simulink model "PubIfDecisionLM_MDL"  (R2020b)
settings: configuration reference "DspaceConfig" (kept outside this file)
PostLoadFcn:
  | if any(exist('dsrtsu_mdlpostloadfcn', 'file') ~= 0), dsrtsu_mdlpostloadfcn('Execute', bdroot); end
InitFcn:
  | , if any(exist('dsmpb_private', 'file') ~= 0), dsmpb_private('dsmpb_mdlclblib', 'Init', bdroot); end,
undefined symbols (not defined in the file or in its folder): OFM_OBJ_FUSIONTYPE_E, OFM_OBJ_MOVINGSTATE_E, OFM_OBJ_ORIENTATION_E, OFM_OBJ_TYPE_E, P_LM_Cyc, P_LM_EMLHistKapRcdBufSize, P_LM_EMLHistTrajBaseDis, P_LM_EMLHistTrajPNum, P_LM_EMLKapCorrMaxThre, P_LM_EMLMinKapThre, P_LM_EMLPathDisDiffThre, P_LM_EMLQuaFiltPar, P_LM_EMLTurnActKapThre, P_LM_EMLValidQuaThre, P_LM_FntPath1Disgap, P_LM_FntPath1MinDis, P_LM_FntPath1Timegap, P_LM_FntPath2Disgap, P_LM_FntPath2MinDis, P_LM_FntPath2Timegap, P_LM_FntPath3Disgap, P_LM_FntPath3MinDis, P_LM_FntPath3Timegap, P_LM_FusBLParFiltP, P_LM_FusEVDifC2Thre, P_LM_FusEVOPath1AllVSLDisThre, P_LM_FusEVOPath1AllVSLLostNumThre, P_LM_FusEVOPath1AllVSLQuaThre, P_LM_FusEVOPath1OTLFacNLC, P_LM_FusOTLQuaThre, P_LM_FusOTLSW, P_LM_FusParC0Index, P_LM_FusParC1Index, P_LM_FusParC2Index, P_LM_FusParC3Index, P_LM_FusVSLQuaThre, P_LM_FusVSLSW, P_LM_FusVSLValidSteerWheerAngThre, P_LM_FusVSLValidVxvThre, P_LM_LaneWidth, P_LM_OTLBufTPInfoEvaFactor, P_LM_OTLObjNum, P_LM_OTLObjSelectAgeThre, P_LM_OTLObjSelectDxAssessVx, P_LM_OTLObjSelectDxThre, P_LM_OTLObjSelectVxThre, P_LM_OTLObjSelectVyAssessDx, P_LM_OTLObjSelectVyThre, P_LM_OTLTrajPntBaseDis, P_LM_OTLTrajStdThre, P_LM_VSLAvailLineNum, P_LM_VSLBLSDiffThre, P_LM_VSLBLSDisRatio, P_LM_VSLFusBLParFiltP_C1, P_LM_VSLFusBLParFiltP_C2, P_LM_VSLFusBLParFiltP_C3, P_LM_VSLFusBLParFiltP_Quality, P_LM_VSLHistTrajBaseDis, P_LM_VSLHistTrajPNum, P_LM_VSLLCC0diff ... (+18)
libraries: simulink x145, LM_LIB x43
(part 23 of 24)

== matlab function PubIfDecisionLM_MDL/Subsystem2/LM_OTL/LM_OTL_MovObjTrajFit/LM_OTL_TrajFit/MATLAB Function3 ==
  data: LM_OTLBufL1DxVect input; LM_OTLBufL1DyVect input; LM_OTLBufL2DxVect input; LM_OTLBufL2DyVect input; LM_OTLBufE1DxVect input; LM_OTLBufE1DyVect input; LM_OTLBufE2DxVect input; LM_OTLBufE2DyVect input; LM_OTLBufR1DxVect input; LM_OTLBufR1DyVect input; LM_OTLBufR2DxVect input; LM_OTLBufR2DyVect input; LM_OTLBufL1SPPos input; LM_OTLBufL2SPPos input; LM_OTLBufE1SPPos input; LM_OTLBufE2SPPos input; LM_OTLBufR1SPPos input; LM_OTLBufR2SPPos input; LM_OTLBufL1LastSPPos input; LM_OTLBufL2LastSPPos input; LM_OTLBufE1LastSPPos input; LM_OTLBufE2LastSPPos input; LM_OTLBufR1LastSPPos input; LM_OTLBufR2LastSPPos input; LM_OTLBufL1PNum input; LM_OTLBufL2PNum input; LM_OTLBufE1PNum input; LM_OTLBufE2PNum input; LM_OTLBufR1PNum input; LM_OTLBufR2PNum input; LM_OTLBufL1LastPNum input; LM_OTLBufL2LastPNum input; LM_OTLBufE1LastPNum input; LM_OTLBufE2LastPNum input; LM_OTLBufR1LastPNum input; LM_OTLBufR2LastPNum input; LM_OTLBufL1Flg input; LM_OTLBufL2Flg input; LM_OTLBufE1Flg input; LM_OTLBufE2Flg input; LM_OTLBufR1Flg input; LM_OTLBufR2Flg input; LM_OTLBufL1LastFlg input; LM_OTLBufL2LastFlg input; LM_OTLBufE1LastFlg input; LM_OTLBufE2LastFlg input; LM_OTLBufR1LastFlg input; LM_OTLBufR2LastFlg input; LM_OTLBufL1Offset input; LM_OTLBufL2Offset input; LM_OTLBufE1Offset input; LM_OTLBufE2Offset input; LM_OTLBufR1Offset input; LM_OTLBufR2Offset input; LM_OTLBufL1LastOffset input; LM_OTLBufL2LastOffset input; LM_OTLBufE1LastOffset input; LM_OTLBufE2LastOffset input; LM_OTLBufR1LastOffset input; LM_OTLBufR2LastOffset input; LM_OTLBufResampeFntPathDxInfo output; LM_OTLBufResampeFntPathDyInfo output
function [LM_OTLBufResampeFntPathDxInfo,LM_OTLBufResampeFntPathDyInfo] = fcn(LM_OTLBufL1DxVect,LM_OTLBufL1DyVect,LM_OTLBufL2DxVect,LM_OTLBufL2DyVect,LM_OTLBufE1DxVect,LM_OTLBufE1DyVect,LM_OTLBufE2DxVect,LM_OTLBufE2DyVect,LM_OTLBufR1DxVect,LM_OTLBufR1DyVect,LM_OTLBufR2DxVect,LM_OTLBufR2DyVect,...
                                                              LM_OTLBufL1SPPos,LM_OTLBufL2SPPos,LM_OTLBufE1SPPos,LM_OTLBufE2SPPos,LM_OTLBufR1SPPos,LM_OTLBufR2SPPos,LM_OTLBufL1LastSPPos,LM_OTLBufL2LastSPPos,LM_OTLBufE1LastSPPos,LM_OTLBufE2LastSPPos,LM_OTLBufR1LastSPPos,LM_OTLBufR2LastSPPos,...
                                                              LM_OTLBufL1PNum,LM_OTLBufL2PNum,LM_OTLBufE1PNum,LM_OTLBufE2PNum,LM_OTLBufR1PNum,LM_OTLBufR2PNum,LM_OTLBufL1LastPNum,LM_OTLBufL2LastPNum,LM_OTLBufE1LastPNum,LM_OTLBufE2LastPNum,LM_OTLBufR1LastPNum,LM_OTLBufR2LastPNum,...
                                                              LM_OTLBufL1Flg,LM_OTLBufL2Flg,LM_OTLBufE1Flg,LM_OTLBufE2Flg,LM_OTLBufR1Flg,LM_OTLBufR2Flg,LM_OTLBufL1LastFlg,LM_OTLBufL2LastFlg,LM_OTLBufE1LastFlg,LM_OTLBufE2LastFlg,LM_OTLBufR1LastFlg,LM_OTLBufR2LastFlg,...
                                                              LM_OTLBufL1Offset,LM_OTLBufL2Offset,LM_OTLBufE1Offset,LM_OTLBufE2Offset,LM_OTLBufR1Offset,LM_OTLBufR2Offset,LM_OTLBufL1LastOffset,LM_OTLBufL2LastOffset,LM_OTLBufE1LastOffset,LM_OTLBufE2LastOffset,LM_OTLBufR1LastOffset,LM_OTLBufR2LastOffset)
                                                               
%第一段车道车道线采样
%初始化基本参数
P_LM_OTLBufResampPNum = uint8(40);
P_LM_OTLBufResampSPPos = single(0);
P_LM_OTLBufResampBaseDis = single(2);
% output initial                                                           
LM_OTLBufResampeFntPathDxInfo = single(zeros(1,80));
LM_OTLBufResampeFntPathDyInfo = single(zeros(1,80));
%初始化各buffer轨迹点索引位置  
t_bufl1index = uint8(0);
t_bufl2index = uint8(0);
t_bufe1index = uint8(0);
t_bufe2index = uint8(0);
t_bufr1index = uint8(0);
t_bufr2index = uint8(0);
t_bufl1lastindex = uint8(0);
t_bufl2lastindex = uint8(0);
t_bufe1lastindex = uint8(0);
t_bufe2lastindex = uint8(0);
t_bufr1lastindex = uint8(0);
t_bufr2lastindex = uint8(0);
%第一段车道车道线采样
for i = 1:P_LM_OTLBufResampPNum
    temp1 = (single(i-1))*P_LM_OTLBufResampBaseDis + P_LM_OTLBufResampSPPos;
    temp2 = (single(i))*P_LM_OTLBufResampBaseDis + P_LM_OTLBufResampSPPos;
    %初始化该区间范围内有效轨迹点个数
    t_tpnum = uint8(0);
    t_tpdxsum = single(0);
    t_tpdysum = single(0);
    %判断BufL1前目标是否存在该区间的轨迹点
    if LM_OTLBufL1LastFlg(1) ~= 0
        if t_bufl1lastindex < LM_OTLBufL1LastPNum(1)
            t_index = t_bufl1lastindex + LM_OTLBufL1LastSPPos(1);
            if t_index > 80
                t_index = t_index - uint8(80);
            end
            t_tpdx = LM_OTLBufL1DxVect(t_index);
            t_tpdy = LM_OTLBufL1DyVect(t_index)-LM_OTLBufL1LastOffset(1);
            if t_tpdx >= temp1  && t_tpdx < temp2
                t_tpnum = t_tpnum +uint8(1);
                t_tpdxsum = t_tpdxsum + t_tpdx;
                t_tpdysum = t_tpdysum + t_tpdy;
                t_bufl1lastindex = t_bufl1lastindex +uint8(1);
            end
        end
    end
    %判断BufL1当前目标是否存在该区间的轨迹点
    if LM_OTLBufL1Flg(1) ~= 0
        if t_bufl1index < LM_OTLBufL1PNum(1)
            t_index = t_bufl1index + LM_OTLBufL1SPPos(1);
            if t_index > 80
                t_index = t_index - uint8(80);
            end
            t_tpdx = LM_OTLBufL1DxVect(t_index);
            t_tpdy = LM_OTLBufL1DyVect(t_index)-LM_OTLBufL1Offset(1);
            if t_tpdx >= temp1  && t_tpdx < temp2
                t_tpnum = t_tpnum +uint8(1);
                t_tpdxsum = t_tpdxsum + t_tpdx;
                t_tpdysum = t_tpdysum + t_tpdy;
                t_bufl1index = t_bufl1index +uint8(1);
            end
        end
    end
    %判断BufL2前目标是否存在该区间的轨迹点
    if LM_OTLBufL2LastFlg(1) ~= 0
        if t_bufl2lastindex < LM_OTLBufL2LastPNum(1)
            t_index = t_bufl2lastindex + LM_OTLBufL2LastSPPos(1);
            if t_index > 80
                t_index = t_index - uint8(80);
            end
            t_tpdx = LM_OTLBufL2DxVect(t_index);
            t_tpdy = LM_OTLBufL2DyVect(t_index)-LM_OTLBufL2LastOffset(1);
            if t_tpdx >= temp1  && t_tpdx < temp2 
                t_tpnum = t_tpnum +uint8(1);
                t_tpdxsum = t_tpdxsum + t_tpdx;
                t_tpdysum = t_tpdysum + t_tpdy;
                t_bufl2lastindex = t_bufl2lastindex +uint8(1);
            end
        end
    end
    %判断BufL2当前目标是否存在该区间的轨迹点
    if LM_OTLBufL2Flg(1) ~= 0
        if t_bufl2index < LM_OTLBufL2PNum(1)
            t_index = t_bufl2index + LM_OTLBufL2SPPos(1);
            if t_index > 80
                t_index = t_index - uint8(80);
            end
            t_tpdx = LM_OTLBufL2DxVect(t_index);
            t_tpdy = LM_OTLBufL2DyVect(t_index)-LM_OTLBufL2Offset(1);
            if t_tpdx >= temp1  && t_tpdx < temp2 
                t_tpnum = t_tpnum +uint8(1);
                t_tpdxsum = t_tpdxsum + t_tpdx;
                t_tpdysum = t_tpdysum + t_tpdy;
                t_bufl2index = t_bufl2index +uint8(1);
            end
        end
    end
    %判断BufE1前目标是否存在该区间的轨迹点
    if LM_OTLBufE1LastFlg(1) ~= 0
        if t_bufe1lastindex < LM_OTLBufE1LastPNum(1)
            t_index = t_bufe1lastindex + LM_OTLBufE1LastSPPos(1);
            if t_index > 80
                t_index = t_index - uint8(80);
            end
            t_tpdx = LM_OTLBufE1DxVect(t_index);
            t_tpdy = LM_OTLBufE1DyVect(t_index)-LM_OTLBufE1LastOffset(1);
            if t_tpdx >= temp1  && t_tpdx < temp2 
                t_tpnum = t_tpnum +uint8(1);
                t_tpdxsum = t_tpdxsum + t_tpdx;
                t_tpdysum = t_tpdysum + t_tpdy;
                t_bufe1lastindex = t_bufe1lastindex +uint8(1);
            end
        end
    end
    %判断BufE1当前目标是否存在该区间的轨迹点
    if LM_OTLBufE1Flg(1) ~= 0
        if t_bufe1index < LM_OTLBufE1PNum(1)
            t_index = t_bufe1index + LM_OTLBufE1SPPos(1);
            if t_index > 80
                t_index = t_index - uint8(80);
            end
            t_tpdx = LM_OTLBufE1DxVect(t_index);
            t_tpdy = LM_OTLBufE1DyVect(t_index)-LM_OTLBufE1Offset(1);
            if t_tpdx >= temp1  && t_tpdx < temp2 
                t_tpnum = t_tpnum +uint8(1);
                t_tpdxsum = t_tpdxsum + t_tpdx;
                t_tpdysum = t_tpdysum + t_tpdy;
                t_bufe1index = t_bufe1index +uint8(1);
            end
        end
    end
    %判断BufE2前目标是否存在该区间的轨迹点
    if LM_OTLBufE2LastFlg(1) ~= 0
        if t_bufe2lastindex < LM_OTLBufE2LastPNum(1)
            t_index = t_bufe2lastindex + LM_OTLBufE2LastSPPos(1);
            if t_index > 80
                t_index = t_index - uint8(80);
            end
            t_tpdx = LM_OTLBufE2DxVect(t_index);
            t_tpdy = LM_OTLBufE2DyVect(t_index)-LM_OTLBufE2LastOffset(1);
            if t_tpdx >= temp1 && t_tpdx < temp2 
                t_tpnum = t_tpnum +uint8(1);
                t_tpdxsum = t_tpdxsum + t_tpdx;
                t_tpdysum = t_tpdysum + t_tpdy;
                t_bufe2lastindex = t_bufe2lastindex +uint8(1);
            end
        end
    end
    %判断BufE2当前目标是否存在该区间的轨迹点
    if LM_OTLBufE2Flg(1) ~= 0
        if t_bufe2index < LM_OTLBufE2PNum(1)
            t_index = t_bufe2index + LM_OTLBufE2SPPos(1);
            if t_index > 80
                t_index = t_index - uint8(80);
            end
            t_tpdx = LM_OTLBufE2DxVect(t_index);
            t_tpdy = LM_OTLBufE2DyVect(t_index)-LM_OTLBufE2Offset(1);
            if t_tpdx >= temp1  && t_tpdx < temp2 
                t_tpnum = t_tpnum +uint8(1);
                t_tpdxsum = t_tpdxsum + t_tpdx;
                t_tpdysum = t_tpdysum + t_tpdy;
                t_bufe2index = t_bufe2index +uint8(1);
            end
        end
    end
    %判断BufR1前目标否存在该区间的轨迹点
    if LM_OTLBufR1LastFlg(1) ~= 0
        if t_bufr1lastindex < LM_OTLBufR1LastPNum(1)
            t_index = t_bufr1lastindex +  LM_OTLBufR1LastSPPos(1);
            if t_index > 80
                t_index = t_index - uint8(80);
            end
            t_tpdx = LM_OTLBufR1DxVect(t_index);
            t_tpdy = LM_OTLBufR1DyVect(t_index)-LM_OTLBufR1LastOffset(1);
            if t_tpdx >= temp1  && t_tpdx < temp2 
                t_tpnum = t_tpnum +uint8(1);
                t_tpdxsum = t_tpdxsum + t_tpdx;
                t_tpdysum = t_tpdysum + t_tpdy;
                t_bufr1lastindex = t_bufr1lastindex +uint8(1);
            end
        end
    end
    %判断BufR1当前目标否存在该区间的轨迹点
    if LM_OTLBufR1Flg(1) ~= 0
        if t_bufr1index < LM_OTLBufR1PNum(1)
            t_index = t_bufr1index +  LM_OTLBufR1SPPos(1);
            if t_index > 80
                t_index = t_index - uint8(80);
            end
            t_tpdx = LM_OTLBufR1DxVect(t_index);
            t_tpdy = LM_OTLBufR1DyVect(t_index)-LM_OTLBufR1Offset(1);
            if t_tpdx >= temp1  && t_tpdx < temp2 
                t_tpnum = t_tpnum +uint8(1);
                t_tpdxsum = t_tpdxsum + t_tpdx;
                t_tpdysum = t_tpdysum + t_tpdy;
                t_bufr1index = t_bufr1index +uint8(1);
            end
        end
    end
    %判断BufR2前目标是否存在该区间的轨迹点
    if LM_OTLBufR2LastFlg(1) ~= 0
        if t_bufr2lastindex < LM_OTLBufR2LastPNum(1)
            t_index = t_bufr2lastindex + LM_OTLBufR2LastSPPos(1);
            if t_index > 80
                t_index = t_index - uint8(80);
            end
            t_tpdx = LM_OTLBufR2DxVect(t_index);
            t_tpdy = LM_OTLBufR2DyVect(t_index)-LM_OTLBufR2LastOffset(1);
            if t_tpdx >= temp1  && t_tpdx < temp2 
                t_tpnum = t_tpnum +uint8(1);
                t_tpdxsum = t_tpdxsum + t_tpdx;
                t_tpdysum = t_tpdysum + t_tpdy;
                t_bufr2lastindex = t_bufr2lastindex +uint8(1);
            end
        end
    end
    %判断BufR2当前目标是否存在该区间的轨迹点
    if LM_OTLBufR2Flg(1) ~= 0
        if t_bufr2index < LM_OTLBufR2PNum(1)
            t_index = t_bufr2index + LM_OTLBufR2SPPos(1);
            if t_index > 80
                t_index = t_index - uint8(80);
            end
            t_tpdx = LM_OTLBufR2DxVect(t_index);
            t_tpdy = LM_OTLBufR2DyVect(t_index)-LM_OTLBufR2Offset(1);
            if t_tpdx >= temp1  && t_tpdx < temp2 
                t_tpnum = t_tpnum +uint8(1);
                t_tpdxsum = t_tpdxsum + t_tpdx;
                t_tpdysum = t_tpdysum + t_tpdy;
                t_bufr2index = t_bufr2index +uint8(1);
            end
        end
    end
    if t_tpnum ~= 0
        t_tpdx = t_tpdxsum / single(t_tpnum);
        t_tpdy = t_tpdysum / single(t_tpnum);
    else
        t_tpdx = single(0);
        t_tpdy = single(0);
    end
    LM_OTLBufResampeFntPathDxInfo(i) = t_tpdx;
    LM_OTLBufResampeFntPathDyInfo(i) = t_tpdy;
end
%第二段车道车道线采样
%初始化基本参数
P_LM_OTLBufResampPNum = uint8(40);
P_LM_OTLBufResampSPPos = single(35);
P_LM_OTLBufResampBaseDis = single(2);
%初始化各buffer轨迹点索引位置  
t_bufl1index = uint8(0);
t_bufl2index = uint8(0);
t_bufe1index = uint8(0);
t_bufe2index = uint8(0);
t_bufr1index = uint8(0);
t_bufr2index = uint8(0);
t_bufl1lastindex = uint8(0);
t_bufl2lastindex = uint8(0);
t_bufe1lastindex = uint8(0);
t_bufe2lastindex = uint8(0);
t_bufr1lastindex = uint8(0);
t_bufr2lastindex = uint8(0);

for i = 1:P_LM_OTLBufResampPNum
    temp1 = (single(i-1))*P_LM_OTLBufResampBaseDis + P_LM_OTLBufResampSPPos;
    temp2 = (single(i))*P_LM_OTLBufResampBaseDis + P_LM_OTLBufResampSPPos;
    %初始化该区间范围内有效轨迹点个数
    t_tpnum = uint8(0);
    t_tpdxsum = single(0);
    t_tpdysum = single(0);
    %判断BufL1前目标是否存在该区间的轨迹点
    if LM_OTLBufL1LastFlg(2) ~= 0
        if t_bufl1lastindex < LM_OTLBufL1LastPNum(2)
            t_index = t_bufl1lastindex + LM_OTLBufL1LastSPPos(2);
            if t_index > 80
                t_index = t_index - uint8(80);
            end
            t_tpdx = LM_OTLBufL1DxVect(t_index);
            t_tpdy = LM_OTLBufL1DyVect(t_index)-LM_OTLBufL1LastOffset(2);
            if t_tpdx >= temp1  && t_tpdx < temp2
                t_tpnum = t_tpnum +uint8(1);
                t_tpdxsum = t_tpdxsum + t_tpdx;
                t_tpdysum = t_tpdysum + t_tpdy;
                t_bufl1lastindex = t_bufl1lastindex +uint8(1);
            end
        end
    end
    %判断BufL1当前目标是否存在该区间的轨迹点
    if LM_OTLBufL1Flg(2) ~= 0
        if t_bufl1index < LM_OTLBufL1PNum(2)
            t_index = t_bufl1index + LM_OTLBufL1SPPos(2);
            if t_index > 80
                t_index = t_index - uint8(80);
            end
            t_tpdx = LM_OTLBufL1DxVect(t_index);
            t_tpdy = LM_OTLBufL1DyVect(t_index)-LM_OTLBufL1Offset(2);
            if t_tpdx >= temp1  && t_tpdx < temp2
                t_tpnum = t_tpnum +uint8(1);
                t_tpdxsum = t_tpdxsum + t_tpdx;
                t_tpdysum = t_tpdysum + t_tpdy;
                t_bufl1index = t_bufl1index +uint8(1);
            end
        end
    end
    %判断BufL2前目标是否存在该区间的轨迹点
    if LM_OTLBufL2LastFlg(2) ~= 0
        if t_bufl2lastindex < LM_OTLBufL2LastPNum(2)
            t_index = t_bufl2lastindex + LM_OTLBufL2LastSPPos(2);
            if t_index > 80
                t_index = t_index - uint8(80);
            end
            t_tpdx = LM_OTLBufL2DxVect(t_index);
            t_tpdy = LM_OTLBufL2DyVect(t_index)-LM_OTLBufL2LastOffset(2);
            if t_tpdx >= temp1  && t_tpdx < temp2 
                t_tpnum = t_tpnum +uint8(1);
                t_tpdxsum = t_tpdxsum + t_tpdx;
                t_tpdysum = t_tpdysum + t_tpdy;
                t_bufl2lastindex = t_bufl2lastindex +uint8(1);
            end
        end
    end
    %判断BufL2当前目标是否存在该区间的轨迹点
    if LM_OTLBufL2Flg(2) ~= 0
        if t_bufl2index < LM_OTLBufL2PNum(2)
            t_index = t_bufl2index + LM_OTLBufL2SPPos(2);
            if t_index > 80
                t_index = t_index - uint8(80);
            end
            t_tpdx = LM_OTLBufL2DxVect(t_index);
            t_tpdy = LM_OTLBufL2DyVect(t_index)-LM_OTLBufL2Offset(2);
            if t_tpdx >= temp1  && t_tpdx < temp2 
                t_tpnum = t_tpnum +uint8(1);
                t_tpdxsum = t_tpdxsum + t_tpdx;
                t_tpdysum = t_tpdysum + t_tpdy;
                t_bufl2index = t_bufl2index +uint8(1);
            end
        end
    end
    %判断BufE1前目标是否存在该区间的轨迹点
    if LM_OTLBufE1LastFlg(2) ~= 0
        if t_bufe1lastindex < LM_OTLBufE1LastPNum(2)
            t_index = t_bufe1lastindex + LM_OTLBufE1LastSPPos(2);
            if t_index > 80
                t_index = t_index - uint8(80);
            end
            t_tpdx = LM_OTLBufE1DxVect(t_index);
            t_tpdy = LM_OTLBufE1DyVect(t_index)-LM_OTLBufE1LastOffset(2);
            if t_tpdx >= temp1  && t_tpdx < temp2 
                t_tpnum = t_tpnum +uint8(1);
                t_tpdxsum = t_tpdxsum + t_tpdx;
                t_tpdysum = t_tpdysum + t_tpdy;
                t_bufe1lastindex = t_bufe1lastindex +uint8(1);
            end
        end
    end
    %判断BufE1当前目标是否存在该区间的轨迹点
    if LM_OTLBufE1Flg(2) ~= 0
        if t_bufe1index < LM_OTLBufE1PNum(2)
            t_index = t_bufe1index + LM_OTLBufE1SPPos(2);
            if t_index > 80
                t_index = t_index - uint8(80);
            end
            t_tpdx = LM_OTLBufE1DxVect(t_index);
            t_tpdy = LM_OTLBufE1DyVect(t_index)-LM_OTLBufE1Offset(2);
            if t_tpdx >= temp1  && t_tpdx < temp2 
                t_tpnum = t_tpnum +uint8(1);
                t_tpdxsum = t_tpdxsum + t_tpdx;
                t_tpdysum = t_tpdysum + t_tpdy;
                t_bufe1index = t_bufe1index +uint8(1);
            end
        end
    end
    %判断BufE2前目标是否存在该区间的轨迹点
    if LM_OTLBufE2LastFlg(2) ~= 0
        if t_bufe2lastindex < LM_OTLBufE2LastPNum(2)
            t_index = t_bufe2lastindex + LM_OTLBufE2LastSPPos(2);
            if t_index > 80
                t_index = t_index - uint8(80);
            end
            t_tpdx = LM_OTLBufE2DxVect(t_index);
            t_tpdy = LM_OTLBufE2DyVect(t_index)-LM_OTLBufE2LastOffset(2);
            if t_tpdx >= temp1 && t_tpdx < temp2 
                t_tpnum = t_tpnum +uint8(1);
                t_tpdxsum = t_tpdxsum + t_tpdx;
                t_tpdysum = t_tpdysum + t_tpdy;
                t_bufe2lastindex = t_bufe2lastindex +uint8(1);
            end
        end
    end
    %判断BufE2当前目标是否存在该区间的轨迹点
    if LM_OTLBufE2Flg(2) ~= 0
        if t_bufe2index < LM_OTLBufE2PNum(2)
            t_index = t_bufe2index + LM_OTLBufE2SPPos(2);
            if t_index > 80
                t_index = t_index - uint8(80);
            end
            t_tpdx = LM_OTLBufE2DxVect(t_index);
            t_tpdy = LM_OTLBufE2DyVect(t_index)-LM_OTLBufE2Offset(2);
            if t_tpdx >= temp1  && t_tpdx < temp2 
                t_tpnum = t_tpnum +uint8(1);
                t_tpdxsum = t_tpdxsum + t_tpdx;
                t_tpdysum = t_tpdysum + t_tpdy;
                t_bufe2index = t_bufe2index +uint8(1);
            end
        end
    end
    %判断BufR1前目标否存在该区间的轨迹点
    if LM_OTLBufR1LastFlg(2) ~= 0
        if t_bufr1lastindex < LM_OTLBufR1LastPNum(2)
            t_index = t_bufr1lastindex +  LM_OTLBufR1LastSPPos(2);
            if t_index > 80
                t_index = t_index - uint8(80);
            end
            t_tpdx = LM_OTLBufR1DxVect(t_index);
            t_tpdy = LM_OTLBufR1DyVect(t_index)-LM_OTLBufR1LastOffset(2);
            if t_tpdx >= temp1  && t_tpdx < temp2 
                t_tpnum = t_tpnum +uint8(1);
                t_tpdxsum = t_tpdxsum + t_tpdx;
                t_tpdysum = t_tpdysum + t_tpdy;
                t_bufr1lastindex = t_bufr1lastindex +uint8(1);
            end
        end
    end
    %判断BufR1当前目标否存在该区间的轨迹点
    if LM_OTLBufR1Flg(2) ~= 0
        if t_bufr1index < LM_OTLBufR1PNum(2)
            t_index = t_bufr1index +  LM_OTLBufR1SPPos(2);
            if t_index > 80
                t_index = t_index - uint8(80);
            end
            t_tpdx = LM_OTLBufR1DxVect(t_index);
            t_tpdy = LM_OTLBufR1DyVect(t_index)-LM_OTLBufR1Offset(2);
            if t_tpdx >= temp1  && t_tpdx < temp2 
                t_tpnum = t_tpnum +uint8(1);
                t_tpdxsum = t_tpdxsum + t_tpdx;
                t_tpdysum = t_tpdysum + t_tpdy;
                t_bufr1index = t_bufr1index +uint8(1);
            end
        end
    end
    %判断BufR2前目标是否存在该区间的轨迹点
    if LM_OTLBufR2LastFlg(2) ~= 0
        if t_bufr2lastindex < LM_OTLBufR2LastPNum(2)
            t_index = t_bufr2lastindex + LM_OTLBufR2LastSPPos(2);
            if t_index > 80
                t_index = t_index - uint8(80);
            end
            t_tpdx = LM_OTLBufR2DxVect(t_index);
            t_tpdy = LM_OTLBufR2DyVect(t_index)-LM_OTLBufR2LastOffset(2);
            if t_tpdx >= temp1  && t_tpdx < temp2 
                t_tpnum = t_tpnum +uint8(1);
                t_tpdxsum = t_tpdxsum + t_tpdx;
                t_tpdysum = t_tpdysum + t_tpdy;
                t_bufr2lastindex = t_bufr2lastindex +uint8(1);
            end
        end
    end
    %判断BufR2当前目标是否存在该区间的轨迹点
    if LM_OTLBufR2Flg(2) ~= 0
        if t_bufr2index < LM_OTLBufR2PNum(2)
            t_index = t_bufr2index + LM_OTLBufR2SPPos(2);
            if t_index > 80
                t_index = t_index - uint8(80);
            end
            t_tpdx = LM_OTLBufR2DxVect(t_index);
            t_tpdy = LM_OTLBufR2DyVect(t_index)-LM_OTLBufR2Offset(2);
            if t_tpdx >= temp1  && t_tpdx < temp2 
                t_tpnum = t_tpnum +uint8(1);
                t_tpdxsum = t_tpdxsum + t_tpdx;
                t_tpdysum = t_tpdysum + t_tpdy;
                t_bufr2index = t_bufr2index +uint8(1);
            end
        end
    end
    if t_tpnum ~= 0
        t_tpdx = t_tpdxsum / single(t_tpnum);
        t_tpdy = t_tpdysum / single(t_tpnum);
    else
        t_tpdx = single(0);
        t_tpdy = single(0);
    end
    if t_tpdx~=0
        index=uint8(ceil(0.5*t_tpdx)+1);
        LM_OTLBufResampeFntPathDxInfo(index) = t_tpdx;
        LM_OTLBufResampeFntPathDyInfo(index) = t_tpdy;
    end
end
%第三段车道车道线采样
%初始化基本参数
P_LM_OTLBufResampPNum = uint8(40);
P_LM_OTLBufResampSPPos = single(70);
P_LM_OTLBufResampBaseDis = single(2);
%初始化各buffer轨迹点索引位置  
t_bufl1index = uint8(0);
t_bufl2index = uint8(0);
t_bufe1index = uint8(0);
t_bufe2index = uint8(0);
t_bufr1index = uint8(0);
t_bufr2index = uint8(0);
t_bufl1lastindex = uint8(0);
t_bufl2lastindex = uint8(0);
t_bufe1lastindex = uint8(0);
t_bufe2lastindex = uint8(0);
t_bufr1lastindex = uint8(0);
t_bufr2lastindex = uint8(0);

for i = 1:P_LM_OTLBufResampPNum
    temp1 = (single(i-1))*P_LM_OTLBufResampBaseDis + P_LM_OTLBufResampSPPos;
    temp2 = (single(i))*P_LM_OTLBufResampBaseDis + P_LM_OTLBufResampSPPos;
    %初始化该区间范围内有效轨迹点个数
    t_tpnum = uint8(0);
    t_tpdxsum = single(0);
    t_tpdysum = single(0);
    %判断BufL1前目标是否存在该区间的轨迹点
    if LM_OTLBufL1LastFlg(3) ~= 0
        if t_bufl1lastindex < LM_OTLBufL1LastPNum(3)
            t_index = t_bufl1lastindex + LM_OTLBufL1LastSPPos(3);
            if t_index > 80
                t_index = t_index - uint8(80);
            end
            t_tpdx = LM_OTLBufL1DxVect(t_index);
            t_tpdy = LM_OTLBufL1DyVect(t_index)-LM_OTLBufL1LastOffset(3);
            if t_tpdx >= temp1  && t_tpdx < temp2
                t_tpnum = t_tpnum +uint8(1);
                t_tpdxsum = t_tpdxsum + t_tpdx;
                t_tpdysum = t_tpdysum + t_tpdy;
                t_bufl1lastindex = t_bufl1lastindex +uint8(1);
            end
        end
    end
    %判断BufL1当前目标是否存在该区间的轨迹点
    if LM_OTLBufL1Flg(3) ~= 0
        if t_bufl1index < LM_OTLBufL1PNum(3)
            t_index = t_bufl1index + LM_OTLBufL1SPPos(3);
            if t_index > 80
                t_index = t_index - uint8(80);
            end
            t_tpdx = LM_OTLBufL1DxVect(t_index);
            t_tpdy = LM_OTLBufL1DyVect(t_index)-LM_OTLBufL1Offset(3);
            if t_tpdx >= temp1  && t_tpdx < temp2
                t_tpnum = t_tpnum +uint8(1);
                t_tpdxsum = t_tpdxsum + t_tpdx;
                t_tpdysum = t_tpdysum + t_tpdy;
                t_bufl1index = t_bufl1index +uint8(1);
            end
        end
    end
    %判断BufL2前目标是否存在该区间的轨迹点
    if LM_OTLBufL2LastFlg(3) ~= 0
        if t_bufl2lastindex < LM_OTLBufL2LastPNum(3)
            t_index = t_bufl2lastindex + LM_OTLBufL2LastSPPos(3);
            if t_index > 80
                t_index = t_index - uint8(80);
            end
            t_tpdx = LM_OTLBufL2DxVect(t_index);
            t_tpdy = LM_OTLBufL2DyVect(t_index)-LM_OTLBufL2LastOffset(3);
            if t_tpdx >= temp1  && t_tpdx < temp2 
                t_tpnum = t_tpnum +uint8(1);
                t_tpdxsum = t_tpdxsum + t_tpdx;
                t_tpdysum = t_tpdysum + t_tpdy;
                t_bufl2lastindex = t_bufl2lastindex +uint8(1);
            end
        end
    end
    %判断BufL2当前目标是否存在该区间的轨迹点
    if LM_OTLBufL2Flg(3) ~= 0
        if t_bufl2index < LM_OTLBufL2PNum(3)
            t_index = t_bufl2index + LM_OTLBufL2SPPos(3);
            if t_index > 80
                t_index = t_index - uint8(80);
            end
            t_tpdx = LM_OTLBufL2DxVect(t_index);
            t_tpdy = LM_OTLBufL2DyVect(t_index)-LM_OTLBufL2Offset(3);
            if t_tpdx >= temp1  && t_tpdx < temp2 
                t_tpnum = t_tpnum +uint8(1);
                t_tpdxsum = t_tpdxsum + t_tpdx;
                t_tpdysum = t_tpdysum + t_tpdy;
                t_bufl2index = t_bufl2index +uint8(1);
            end
        end
    end
    %判断BufE1前目标是否存在该区间的轨迹点
    if LM_OTLBufE1LastFlg(3) ~= 0
        if t_bufe1lastindex < LM_OTLBufE1LastPNum(3)
            t_index = t_bufe1lastindex + LM_OTLBufE1LastSPPos(3);
            if t_index > 80
                t_index = t_index - uint8(80);
            end
            t_tpdx = LM_OTLBufE1DxVect(t_index);
            t_tpdy = LM_OTLBufE1DyVect(t_index)-LM_OTLBufE1LastOffset(3);
            if t_tpdx >= temp1  && t_tpdx < temp2 
                t_tpnum = t_tpnum +uint8(1);
                t_tpdxsum = t_tpdxsum + t_tpdx;
                t_tpdysum = t_tpdysum + t_tpdy;
                t_bufe1lastindex = t_bufe1lastindex +uint8(1);
            end
        end
    end
    %判断BufE1当前目标是否存在该区间的轨迹点
    if LM_OTLBufE1Flg(3) ~= 0
        if t_bufe1index < LM_OTLBufE1PNum(3)
            t_index = t_bufe1index + LM_OTLBufE1SPPos(3);
            if t_index > 80
                t_index = t_index - uint8(80);
            end
            t_tpdx = LM_OTLBufE1DxVect(t_index);
            t_tpdy = LM_OTLBufE1DyVect(t_index)-LM_OTLBufE1Offset(3);
            if t_tpdx >= temp1  && t_tpdx < temp2 
                t_tpnum = t_tpnum +uint8(1);
                t_tpdxsum = t_tpdxsum + t_tpdx;
                t_tpdysum = t_tpdysum + t_tpdy;
                t_bufe1index = t_bufe1index +uint8(1);
            end
        end
    end
    %判断BufE2前目标是否存在该区间的轨迹点
    if LM_OTLBufE2LastFlg(3) ~= 0
        if t_bufe2lastindex < LM_OTLBufE2LastPNum(3)
            t_index = t_bufe2lastindex + LM_OTLBufE2LastSPPos(3);
            if t_index > 80
                t_index = t_index - uint8(80);
            end
            t_tpdx = LM_OTLBufE2DxVect(t_index);
            t_tpdy = LM_OTLBufE2DyVect(t_index)-LM_OTLBufE2LastOffset(3);
            if t_tpdx >= temp1 && t_tpdx < temp2 
                t_tpnum = t_tpnum +uint8(1);
                t_tpdxsum = t_tpdxsum + t_tpdx;
                t_tpdysum = t_tpdysum + t_tpdy;
                t_bufe2lastindex = t_bufe2lastindex +uint8(1);
            end
        end
    end
    %判断BufE2当前目标是否存在该区间的轨迹点
    if LM_OTLBufE2Flg(3) ~= 0
        if t_bufe2index < LM_OTLBufE2PNum(3)
            t_index = t_bufe2index + LM_OTLBufE2SPPos(3);
            if t_index > 80
                t_index = t_index - uint8(80);
            end
            t_tpdx = LM_OTLBufE2DxVect(t_index);
            t_tpdy = LM_OTLBufE2DyVect(t_index)-LM_OTLBufE2Offset(3);
            if t_tpdx >= temp1  && t_tpdx < temp2 
                t_tpnum = t_tpnum +uint8(1);
                t_tpdxsum = t_tpdxsum + t_tpdx;
                t_tpdysum = t_tpdysum + t_tpdy;
                t_bufe2index = t_bufe2index +uint8(1);
            end
        end
    end
    %判断BufR1前目标否存在该区间的轨迹点
    if LM_OTLBufR1LastFlg(3) ~= 0
        if t_bufr1lastindex < LM_OTLBufR1LastPNum(3)
            t_index = t_bufr1lastindex +  LM_OTLBufR1LastSPPos(3);
            if t_index > 80
                t_index = t_index - uint8(80);
            end
            t_tpdx = LM_OTLBufR1DxVect(t_index);
            t_tpdy = LM_OTLBufR1DyVect(t_index)-LM_OTLBufR1LastOffset(3);
            if t_tpdx >= temp1  && t_tpdx < temp2 
                t_tpnum = t_tpnum +uint8(1);
                t_tpdxsum = t_tpdxsum + t_tpdx;
                t_tpdysum = t_tpdysum + t_tpdy;
                t_bufr1lastindex = t_bufr1lastindex +uint8(1);
            end
        end
    end
    %判断BufR1当前目标否存在该区间的轨迹点
    if LM_OTLBufR1Flg(3) ~= 0
        if t_bufr1index < LM_OTLBufR1PNum(3)
            t_index = t_bufr1index +  LM_OTLBufR1SPPos(3);
            if t_index > 80
                t_index = t_index - uint8(80);
            end
            t_tpdx = LM_OTLBufR1DxVect(t_index);
            t_tpdy = LM_OTLBufR1DyVect(t_index)-LM_OTLBufR1Offset(3);
            if t_tpdx >= temp1  && t_tpdx < temp2 
                t_tpnum = t_tpnum +uint8(1);
                t_tpdxsum = t_tpdxsum + t_tpdx;
                t_tpdysum = t_tpdysum + t_tpdy;
                t_bufr1index = t_bufr1index +uint8(1);
            end
        end
    end
    %判断BufR2前目标是否存在该区间的轨迹点
    if LM_OTLBufR2LastFlg(3) ~= 0
        if t_bufr2lastindex < LM_OTLBufR2LastPNum(3)
            t_index = t_bufr2lastindex + LM_OTLBufR2LastSPPos(3);
            if t_index > 80
                t_index = t_index - uint8(80);
            end
            t_tpdx = LM_OTLBufR2DxVect(t_index);
            t_tpdy = LM_OTLBufR2DyVect(t_index)-LM_OTLBufR2LastOffset(3);
            if t_tpdx >= temp1  && t_tpdx < temp2 
                t_tpnum = t_tpnum +uint8(1);
                t_tpdxsum = t_tpdxsum + t_tpdx;
                t_tpdysum = t_tpdysum + t_tpdy;
                t_bufr2lastindex = t_bufr2lastindex +uint8(1);
            end
        end
    end
    %判断BufR2当前目标是否存在该区间的轨迹点
    if LM_OTLBufR2Flg(3) ~= 0
        if t_bufr2index < LM_OTLBufR2PNum(3)
            t_index = t_bufr2index + LM_OTLBufR2SPPos(3);
            if t_index > 80
                t_index = t_index - uint8(80);
            end
            t_tpdx = LM_OTLBufR2DxVect(t_index);
            t_tpdy = LM_OTLBufR2DyVect(t_index)-LM_OTLBufR2Offset(3);
            if t_tpdx >= temp1  && t_tpdx < temp2 
                t_tpnum = t_tpnum +uint8(1);
                t_tpdxsum = t_tpdxsum + t_tpdx;
                t_tpdysum = t_tpdysum + t_tpdy;
                t_bufr2index = t_bufr2index +uint8(1);
            end
        end
    end
    if t_tpnum ~= 0
        t_tpdx = t_tpdxsum / single(t_tpnum);
        t_tpdy = t_tpdysum / single(t_tpnum);
    else
        t_tpdx = single(0);
        t_tpdy = single(0);
    end
    if t_tpdx ~=0
        index=uint8(ceil(0.5*t_tpdx)+2);
        LM_OTLBufResampeFntPathDxInfo(index) = t_tpdx;
        LM_OTLBufResampeFntPathDyInfo(index) = t_tpdy;
    end
end
end

== stateflow chart PubIfDecisionLM_MDL/Subsystem2/LM_SigPrePro1/Subsystem1/LM_RFMLineInfoFilter/Chart1 ==
  state Lost
    en:LM_LINE_Filt = RFM_LINE;
    du:LM_LINE_Filt = RFM_LINE;
    ex:LM_LINE_Filt = LM_LINE_K1;
  state filt
    en:LM_LINE_Filt = LM_LINE_K1;
    existimes = uint8(0);
    du:
    existimes = existimes +uint8(1);
    LM_LINE_Filt = LM_LINE_K1;
    ex:LM_LINE_Filt = LM_LINE_K1;
  state Exist
    en:
    if abs(RFM_LINE.dC2V) <= 0.25 && abs(RFM_LINE.dC3V) <= 1 && abs(RFM_LINE.dC1V) <= 1
    LM_LINE_Filt = RFM_LINE；
    else
    LM_LINE_Filt = LM_LINE_K1;
    end
    du:
    if abs(RFM_LINE.dC2V) <= 0.25 && abs(RFM_LINE.dC3V) <= 1 && abs(RFM_LINE.dC1V) <= 1
    LM_LINE_Filt = RFM_LINE；
    if abs(RFM_LINE.dC2V-LM_LINE_K1.dC2V) <= 1 &&  abs(RFM_LINE.dC3V-LM_LINE_K1.dC3V) <= 1
    LM_LINE_Filt.dC0V=LM_LINE_K1.dC0V+0.75*(RFM_LINE.dC0V-LM_LINE_K1.dC0V);
    LM_LINE_Filt.dC1V=LM_LINE_K1.dC1V+0.75*(RFM_LINE.dC1V-LM_LINE_K1.dC1V);
    LM_LINE_Filt.dC2V=LM_LINE_K1.dC2V+0.15*(RFM_LINE.dC2V-LM_LINE_K1.dC2V);
    LM_LINE_Filt.dC3V=LM_LINE_K1.dC3V+0.15*(RFM_LINE.dC3V-LM_LINE_K1.dC3V);
    LM_LINE_Filt.dDisFront=LM_LINE_K1.dDisFront+0.15*(RFM_LINE.dDisFront-LM_LINE_K1.dDisFront);
    end
    else
    LM_LINE_Filt = LM_LINE_K1;
    end
  (default) -> Lost
  Lost -> filt : [RFM_LINE.bIsLineExist==2]
  Exist -> Lost : [RFM_LINE.bIsLineExist==1]
  filt -> Exist : [RFM_LINE.dQuality >= 0.1 && RFM_LINE.bIsLineExist==2 && existimes >25]
  data: RFM_LINE input Bus: RFM_LINE_BUS; LM_LINE_Filt output Bus: RFM_LINE_BUS size=1; LM_LINE_K1 input Bus: RFM_LINE_BUS; existimes local uint8

== stateflow chart PubIfDecisionLM_MDL/Subsystem2/LM_SigPrePro1/Subsystem1/LM_RFMLineInfoFilter/Chart2 ==
  state Lost
    en:LM_LINE_Filt = RFM_LINE;
    du:LM_LINE_Filt = RFM_LINE;
    ex:LM_LINE_Filt = LM_LINE_K1;
  state filt
    en:LM_LINE_Filt = LM_LINE_K1;
    existimes = uint8(0);
    du:
    existimes = existimes +uint8(1);
    LM_LINE_Filt = LM_LINE_K1;
    ex:LM_LINE_Filt = LM_LINE_K1;
  state Exist
    en:
    if abs(RFM_LINE.dC2V) <= 0.25 && abs(RFM_LINE.dC3V) <= 1 && abs(RFM_LINE.dC1V) <= 1
    LM_LINE_Filt = RFM_LINE；
    else
    LM_LINE_Filt = LM_LINE_K1;
    end
    du:
    if abs(RFM_LINE.dC2V) <= 0.25 && abs(RFM_LINE.dC3V) <= 1 && abs(RFM_LINE.dC1V) <= 1
    LM_LINE_Filt = RFM_LINE；
    if abs(RFM_LINE.dC2V-LM_LINE_K1.dC2V) <= 1 &&  abs(RFM_LINE.dC3V-LM_LINE_K1.dC3V) <= 1
    LM_LINE_Filt.dC0V=LM_LINE_K1.dC0V+0.75*(RFM_LINE.dC0V-LM_LINE_K1.dC0V);
    LM_LINE_Filt.dC1V=LM_LINE_K1.dC1V+0.75*(RFM_LINE.dC1V-LM_LINE_K1.dC1V);
    LM_LINE_Filt.dC2V=LM_LINE_K1.dC2V+0.15*(RFM_LINE.dC2V-LM_LINE_K1.dC2V);
    LM_LINE_Filt.dC3V=LM_LINE_K1.dC3V+0.15*(RFM_LINE.dC3V-LM_LINE_K1.dC3V);
    LM_LINE_Filt.dDisFront=LM_LINE_K1.dDisFront+0.15*(RFM_LINE.dDisFront-LM_LINE_K1.dDisFront);
    end
    else
    LM_LINE_Filt = LM_LINE_K1;
    end
  (default) -> Lost
  Lost -> filt : [RFM_LINE.bIsLineExist==2]
  Exist -> Lost : [RFM_LINE.bIsLineExist==1]
  filt -> Exist : [RFM_LINE.dQuality >= 0.1 && RFM_LINE.bIsLineExist==2 && existimes >25]
  data: RFM_LINE input Bus: RFM_LINE_BUS; LM_LINE_Filt output Bus: RFM_LINE_BUS size=1; LM_LINE_K1 input Bus: RFM_LINE_BUS; existimes local uint8

== stateflow chart PubIfDecisionLM_MDL/Subsystem2/DIR/DrivingIntentionRecognition1/DIR_LaneChangeProbCalc/DIR_LaneChangeLeftProbCalc/Chart ==
  state DIR_LCFalse
    en:
    DIR_LCValid = false;
    du:
    DIR_LCValid = false;
  state DIR_LCMidState2False
    en:
    t_times = uint8(0);
    DIR_LCValid == true;
    du:
    DIR_LCValid == true;
    if SteerWheelAngle < 10
    t_times = t_times + uint8(1);
    else
    t_times = uint8(0);
    end
  state DIR_LCMidState2True
    en:
    t_times = uint8(0);
    DIR_LCValid = false;
    du:
    t_times = t_times + uint8(1);
    DIR_LCValid = false;
  state DIR_LCTure
    en:
    DIR_LCValid = true;
    du:
    DIR_LCValid = true;
  (default) -> DIR_LCFalse
  DIR_LCMidState2False -> DIR_LCFalse [order 2] : [DIR_tLCValid == false && (t_times > uint8(10) || LM_VSLFntPathBaseC1 > 0)]
  DIR_LCFalse -> DIR_LCMidState2True : [DIR_tLCValid == true]
  DIR_LCMidState2True -> DIR_LCFalse [order 1] : [DIR_tLCValid == false]
  DIR_LCMidState2True -> DIR_LCTure [order 2] : [DIR_tLCValid == true && t_times >= uint8(10)]
  DIR_LCMidState2False -> DIR_LCTure [order 1] : [DIR_tLCValid == true]
  DIR_LCTure -> DIR_LCMidState2False : [DIR_tLCValid == false ]
  data: DIR_tLCValid input; SteerWheelAngle input; DIR_LCValid output boolean size=1; t_times local uint8 size=1; LM_VSLFntPathBaseC1 input

== stateflow chart PubIfDecisionLM_MDL/Subsystem2/DIR/DrivingIntentionRecognition1/DIR_LaneChangeProbCalc/DIR_LaneChangeRightProbCalc/Chart1 ==
  state DIR_LCFalse
    en:
    DIR_LCValid = false;
    du:
    DIR_LCValid = false;
  state DIR_LCMidState2False
    en:
    t_times = uint8(0);
    DIR_LCValid == true;
    du:
    DIR_LCValid == true;
    if SteerWheelAngle < 10
    t_times = t_times + uint8(1);
    else
    t_times = uint8(0);
    end
  state DIR_LCMidState2True
    en:
    t_times = uint8(0);
    DIR_LCValid = false;
    du:
    t_times = t_times + uint8(1);
    DIR_LCValid = false;
  state DIR_LCTure
    en:
    DIR_LCValid = true;
    du:
    DIR_LCValid = true;
  (default) -> DIR_LCFalse
  DIR_LCMidState2False -> DIR_LCFalse [order 2] : [DIR_tLCValid == false && (t_times > uint8(10) || LM_VSLFntPathBaseC1 < 0)]
  DIR_LCFalse -> DIR_LCMidState2True : [DIR_tLCValid == true]
  DIR_LCMidState2True -> DIR_LCFalse [order 1] : [DIR_tLCValid == false]
  DIR_LCMidState2True -> DIR_LCTure [order 2] : [DIR_tLCValid == true && t_times >= uint8(10)]
  DIR_LCMidState2False -> DIR_LCTure [order 1] : [DIR_tLCValid == true]
  DIR_LCTure -> DIR_LCMidState2False : [DIR_tLCValid == false ]
  data: DIR_tLCValid input; SteerWheelAngle input; DIR_LCValid output boolean size=1; t_times local uint8 size=1; LM_VSLFntPathBaseC1 input

== stateflow chart PubIfDecisionLM_MDL/Subsystem2/LM_ComFcnProcess/LM_DrivInWLJudge ==
  state UnknowDrivInWL
    en:LM_DrivInWLType=uint8(0);
    du:LM_DrivInWLType=uint8(0);
  state LBExistAndInLeftMost
    en:LM_DrivInWLType=uint8(0);
    REExist_times=uint8(0);
    du:REExist_times=REExist_times+1;
    LM_DrivInWLType=uint8(0);
    ex:REExist_times=uint8(0);
  state RBExist
    en:LM_DrivInWLType=uint8(0);
    REExist_times=uint8(0);
    du:REExist_times=REExist_times+1;
    LM_DrivInWLType=uint8(0);
    ex:REExist_times=uint8(0);
  state LBLost
    en:LM_DrivInWLType= uint8(1);
    RELost_times= uint8(0);
    steertimes= uint8(0);
    REPreDis = single(70);
    du:
    RELost_times=RELost_times+1;
    LM_DrivInWLType= uint8(1);
    if  abs(psiDtOpt) > 0.01
    steertimes = steertimes+1;
    else
    if steertimes==0
    steertimes=uint8(0)；
    else
    steertimes=uint8(steertimes-1);
    end
    end
    REPreDis = REPreDis - vxvRefMs*0.02;
    ex:RELost_times=uint8(0);
  state RBLost
    en:LM_DrivInWLType=uint8(3);
    RELost_times=uint8(0);
    steertimes=uint8(0);
    REPreDis = single(70);
    du:
    RELost_times=RELost_times+1;
    LM_DrivInWLType=uint8(3);
    if  abs(psiDtOpt) > 0.01
    steertimes = steertimes+1;
    else
    if steertimes==0
    steertimes=uint8(0)；
    else
    steertimes=steertimes-1;
    end
    end
    REPreDis = REPreDis - vxvRefMs*0.02;
    ex:RELost_times=uint8(0);
  state DrivInRightMost
    en:LM_DrivInWLType=uint8(3);
    du:LM_DrivInWLType=uint8(3);
  state DrivInLeftMost
    en:LM_DrivInWLType=uint8(1);
    du:LM_DrivInWLType=uint8(1);
  state LBExistButNotInLeftMost
    en:LM_DrivInWLType=uint8(1);
    REOut_times=uint8(0);
    steertimes=uint8(0);
    du:
    REOut_times=REOut_times+1;
    LM_DrivInWLType=uint8(1);
    if  abs(psiDtOpt) > 0.01
    steertimes = steertimes+1;
    else
    if steertimes==0
    steertimes=uint8(0)；
    else
    steertimes=steertimes-1;
    end
    end
    ex:REOut_times= uint8(0);
  state RBExistButNotOutRightMost
    en:LM_DrivInWLType=uint8(3);
    REOut_times=uint8(0);
    steertimes=uint8(0);
    du:
    REOut_times=REOut_times+1;
    LM_DrivInWLType= uint8(3);
    if  abs(psiDtOpt) > 0.01
    steertimes = steertimes+1;
    else
    if steertimes==0
    steertimes=uint8(0)；
    else
    steertimes=steertimes-1;
    end
    end
    ex:REOut_times=uint8(0);
  (default) -> UnknowDrivInWL
  UnknowDrivInWL -> LBExistAndInLeftMost [order 1] : [LM_LBbIsLineExist==2&&LM_LBdC0V<=P_LM_LaneWidth+0.5&&LM_LBdDisStart<=10&&...
      | NumOfLaneDrvDir > 2 ]
  UnknowDrivInWL -> RBExist [order 2] : [LM_RBbIsLineExist==2&&abs(LM_RBdC0V)<=P_LM_LaneWidth+0.5&&LM_RBdDisStart<=10&&...
      | NumOfLaneDrvDir > 2 ]
  RBExist -> UnknowDrivInWL [order 1] : [LM_RBbIsLineExist~=2||abs(LM_RBdC0V)>P_LM_LaneWidth+0.5]
  LBExistAndInLeftMost -> UnknowDrivInWL [order 1] : [LM_LBbIsLineExist~=2||LM_LBdC0V>P_LM_LaneWidth+0.5]
  LBLost -> UnknowDrivInWL [order 2] : [REPreDis<=5 || steertimes >75]
  RBLost -> UnknowDrivInWL [order 2] : [REPreDis<=5 || steertimes >75]
  LBExistButNotInLeftMost -> UnknowDrivInWL [order 1] : [(REOut_times>=25 || steertimes >50)&&...
      | NumOfLaneDrvDir > 2]
  RBExistButNotOutRightMost -> UnknowDrivInWL : [(REOut_times>=25 || steertimes >50)&&...
      | NumOfLaneDrvDir > 2]
  LBExistAndInLeftMost -> DrivInLeftMost [order 2] : [LM_LBbIsLineExist==2&&LM_LBdC0V<=P_LM_LaneWidth+0.5&&LM_LBbIsLineExist==2&&...
      | LM_LBdC0V<=P_LM_LaneWidth+0.5&&LM_LBdDisStart<=10&&REExist_times>=25]
  RBExist -> DrivInRightMost [order 2] : [LM_RBbIsLineExist==2&&abs(LM_RBdC0V)<=P_LM_LaneWidth+0.5&&LM_RBdDisStart<=10&&...
      | NumOfLaneDrvDir > 2 && REExist_times>=25]
  DrivInRightMost -> RBLost [order 1] : [LM_RBbIsLineExist~=2]
  RBLost -> DrivInRightMost [order 1] : [LM_RBbIsLineExist==2&&LM_RBdC0V<=P_LM_LaneWidth+0.5&&...
      | LM_RBdDisStart<=5&&NumOfLaneDrvDir > 1]
  DrivInLeftMost -> LBLost [order 1] : [LM_LBbIsLineExist~=2]
  LBLost -> DrivInLeftMost [order 1] : [LM_LBbIsLineExist==2&&LM_LBdC0V<=P_LM_LaneWidth+0.5&&...
      | LM_LBdDisStart<=10&&NumOfLaneDrvDir > 1]
  DrivInRightMost -> RBExistButNotOutRightMost [order 2] : [LM_LBbIsLineExist==2&&abs(LM_RBdC0V)>P_LM_LaneWidth+0.5&&...
      | LM_LBdDisStart<=10&&NumOfLaneDrvDir > 1]
  LBExistButNotInLeftMost -> DrivInLeftMost [order 2] : [LM_LBbIsLineExist==2&&LM_LBdC0V<=P_LM_LaneWidth+0.5&&...
      | LM_LBdDisStart<=5&&NumOfLaneDrvDir > 2]
  DrivInLeftMost -> LBExistButNotInLeftMost [order 2] : [LM_LBbIsLineExist==2&&LM_LBdC0V>P_LM_LaneWidth+0.5&&...
      | LM_LBdDisStart<=5&&NumOfLaneDrvDir > 1]
  data: LM_L2bIsLineExist input; LM_L2dC0V input; LM_R2bIsLineExist input; LM_R2dC0V input; LM_L1bIsLineExist input; LM_L1eLineType input; LM_R1bIsLineExist input; LM_R1eLineType input; LM_LBbIsLineExist input; LM_LBdC0V input; LM_LBdDisStart input; LM_RBbIsLineExist input; LM_RBdC0V input; LM_RBdDisStart input; NumOfLaneDrvDir input; DrivingOnHighWay input; P_LM_LaneWidth parameter; LM_DrivInWLType output uint8 size=1; REExist_times local uint8; RELost_times local uint8; psiDtOpt input; steertimes local uint8; vxvRefMs input; REPreDis local single size=1; REOut_times local uint8

== matlab function PubIfDecisionLM_MDL/Subsystem2/LM_EML/LM_EMLRearPath1/LM_EMLHistTrajRecordBufferUpdate/MATLAB Function ==
  data: LM_EMLHistPEndPos input; LM_EMLHistTrajVectX output; LM_EMLHistTrajVectXK1Adju input
function LM_EMLHistTrajVectX = fcn(LM_EMLHistPEndPos,LM_EMLHistTrajVectXK1Adju)

LM_EMLHistTrajVectX = LM_EMLHistTrajVectXK1Adju;
LM_EMLHistTrajVectX(LM_EMLHistPEndPos) = single(0);

== matlab function PubIfDecisionLM_MDL/Subsystem2/LM_EML/LM_EMLRearPath1/LM_EMLHistTrajRecordBufferUpdate/MATLAB Function1 ==
  data: LM_EMLHistPEndPos input; LM_EMLHistTrajVectX output; LM_EMLHistTrajVectXK1Adju input
function LM_EMLHistTrajVectX = fcn(LM_EMLHistPEndPos,LM_EMLHistTrajVectXK1Adju)

LM_EMLHistTrajVectX = LM_EMLHistTrajVectXK1Adju;
LM_EMLHistTrajVectX(LM_EMLHistPEndPos) = single(0);
